simulink model "TVC_FSFB_model"  (R2024b)
settings: Solver=ode8  StartTime=0.0  StopTime=60  FixedStep=0.001  RelTol=1e-3
values from neighbouring files (symbols this model uses):
  A = sys_open_loop.A    [LQI_Heavy_STeVe.m]    (also in LQR_Heavy_STeVe.m)
  A_plant = [-d1 0 1; 0 0 1; d3 0 d4]    [LQI_Heavy_STeVe.m]    (also in LQR_Heavy_STeVe.m = [-d1  0   1)
  B = sys_open_loop.B    [LQI_Heavy_STeVe.m]    (also in LQR_Heavy_STeVe.m)
  B_plant = [-d5; 0; d2]    [LQI_Heavy_STeVe.m]    (also in LQR_Heavy_STeVe.m = [-d5)
  K_lqr = lqr(A, B, Q, R)    [LQI_Heavy_STeVe.m]    (also in LQR_Heavy_STeVe.m)
libraries: simulink_extras x5, aerolibactuator x1
settings Model: Creator=jonno  LastModifiedBy=jonno

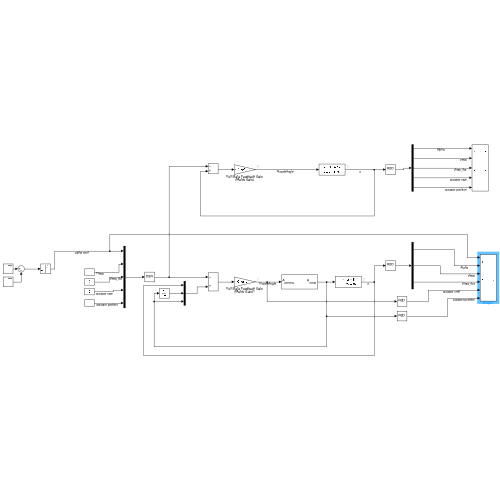
[thumbnail: Simulink's stored preview of the top-level diagram]
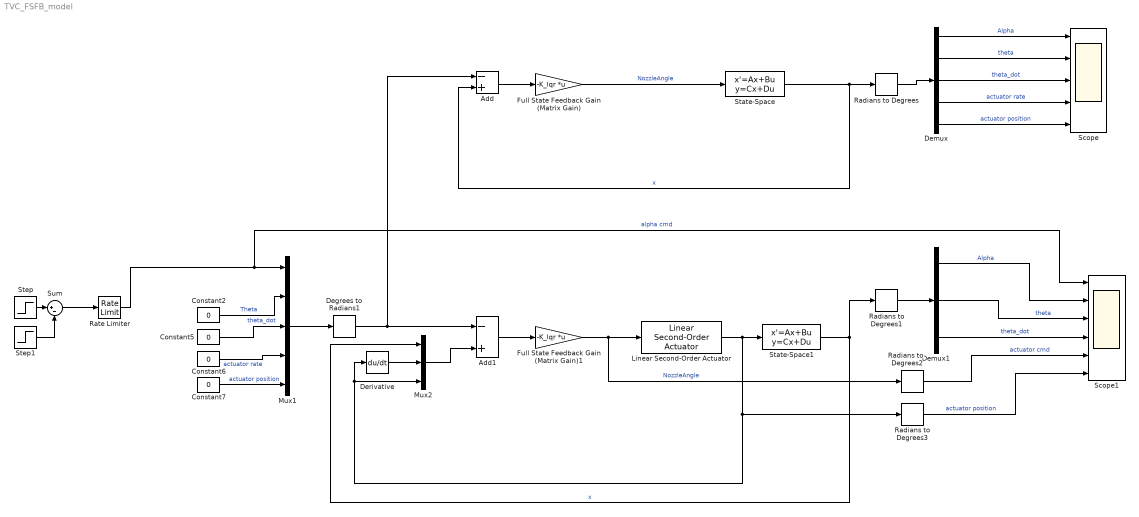
== system TVC_FSFB_model ==
  Add : Sum  Inputs=-+
  Add1 : Sum  Inputs=-+
  Constant{2,5..7} (4 alike) : Constant  Value=0
  Degrees to Radians1 : simulink_extras/Transformations/Degrees to Radians
  Demux : Demux  Outputs=5
  Demux1 : Demux  Outputs=3
  Derivative : Derivative
  Full State Feedback Gain (Matrix Gain) : Gain  Gain=-K_lqr  Multiplication=Matrix(K*u)
  Full State Feedback Gain (Matrix Gain)1 : Gain  Gain=-K_lqr  Multiplication=Matrix(K*u)
  Linear Second-Order Actuator : aerolibactuator/Linear Second-Order Actuator  wn_fin=62  z_fin=0.5858  fin_act_0=0  fin_act_vel=0
  Mux1 : Mux  Inputs=5
  Mux2 : Mux  Inputs=3
  Radians to Degrees{,1..3} (4 alike) : simulink_extras/Transformations/Radians to Degrees
  Rate Limiter : RateLimiter  RisingSlewLimit=0.4  FallingSlewLimit=-0.4  SampleTimeMode=inherited
  Scope : Scope  NumInputPorts=5
  Scope1 : Scope  NumInputPorts=6
  State-Space : StateSpace  A=A  B=B  C=eye(size(A,1))  D=zeros(size(A,1), size(B,2))  InitialCondition=[0 0 0 0 0]
  State-Space1 : StateSpace  A=A_plant  B=B_plant  C=eye(size(A_plant,1))  D=zeros(size(A_plant,1), size(B_plant,2))  InitialCondition=zeros(1, size(A_plant, 2))
  Step : Step  After=10  SampleTime=0
  Step1 : Step  Time=15  After=10  SampleTime=0
  Sum : Sum  Inputs=|+-
  wires:
  Full State Feedback Gain (Matrix Gain)/1 -> State-Space/1  "NozzleAngle"
  State-Space/1 -> Radians to Degrees/1, Add/2  "x"
  Add/1 -> Full State Feedback Gain (Matrix Gain)/1
  Demux/1 -> Scope/1  "Alpha"
  Demux/3 -> Scope/3  "theta_dot"
  Demux/4 -> Scope/4  "actuator rate"
  Demux/2 -> Scope/2  "theta"
  Demux/5 -> Scope/5  "actuator position"
  Radians to Degrees/1 -> Demux/1
  Demux1/2 -> Scope1/3  "theta"
  Degrees to Radians1/1 -> Add/1, Add1/1
  Mux1/1 -> Degrees to Radians1/1
  Constant7/1 -> Mux1/5  "actuator position"
  Constant6/1 -> Mux1/4  "actuator rate"
  Add1/1 -> Full State Feedback Gain (Matrix Gain)1/1
  Full State Feedback Gain (Matrix Gain)1/1 -> Linear Second-Order Actuator/1, Radians to Degrees2/1  "NozzleAngle"
  Constant5/1 -> Mux1/3  "theta_dot"
  State-Space1/1 -> Mux2/1, Radians to Degrees1/1  "x"
  Demux1/1 -> Scope1/2  "Alpha"
  Demux1/3 -> Scope1/4  "theta_dot"
  Radians to Degrees3/1 -> Scope1/6  "actuator position"
  Radians to Degrees1/1 -> Demux1/1
  Mux2/1 -> Add1/2
  Linear Second-Order Actuator/1 -> Radians to Degrees3/1, Mux2/3, Derivative/1, State-Space1/1
  Derivative/1 -> Mux2/2
  Radians to Degrees2/1 -> Scope1/5  "actuator cmd"
  Constant2/1 -> Mux1/2  "Theta"
  Sum/1 -> Rate Limiter/1
  Step/1 -> Sum/1
  Step1/1 -> Sum/2
  Rate Limiter/1 -> Scope1/1, Mux1/1  "alpha cmd"
